simulink model "sldemo_mdlref_datamngt"  (R2019b)
settings: Solver=FixedStepDiscrete  StartTime=0.0  StopTime=10.0  RelTol=1e-3
PreLoadFcn:
  | sldemo_mdlref_datamngt_wsdata
  | sldemo_mdlref_counter_datamngt_types
undefined symbols (not defined in the file): CounterICs, CounterParams
settings Model: ModifiedByFormat=The MathWorks Inc.  ExtModeAutoUpdateStatusClock=off  Creator=The MathWorks, Inc.  LastModifiedBy=The MathWorks Inc.
settings DataIOCC: LimitDataPoints=on  SaveFormat=StructureWithTime  SaveOutput=off  SignalLogging=off  DSMLogging=off  SaveTime=off  ReturnWorkspaceOutputs=off  SignalLoggingName=logsOut
settings OptimizationCC: DefaultParameterBehavior=Inlined  InlineInvariantSignals=on  EnhancedBackFolding=on  StrengthReduction=on  ExpressionDepthLimit=2147483647  StateBitsets=on  DataBitsets=on  EfficientFloat2IntCast=on  LifeSpan=inf
settings DebuggingCC: SaveWithParameterizedLinksMsg=none  CheckExecutionContextPreStartOutputMsg=on  CheckExecutionContextRuntimeOutputMsg=on  MultiTaskDSMMsg=warning  MultiTaskCondExecSysMsg=none  SigSpecEnsureSampleTimeMsg=none  FcnCallInpInsideContextMsg=warning  StateNameClashWarn=warning  StrictBusMsg=ErrorOnBusTreatedAsVector  SFUnexpectedBacktrackingDiag=warning  SFNoUnconditionalDefaultTransitionDiag=warning  SFExecutionAtInitializationDiag=none  ArithmeticOperatorsInVariantConditions=warning
settings HardwareCC: ProdBitPerPointer=32  ProdBitPerSizeT=32  ProdBitPerPtrDiffT=32  ProdLargestAtomicFloat=None  ProdIntDivRoundTo=Undefined  ProdEndianess=Unspecified  ProdWordSize=32  ProdHWDeviceType=32-bit Generic  TargetHWDeviceType=32-bit Generic
settings ModelReferenceCC: UpdateModelReferenceTargets=IfOutOfDate  CheckModelReferenceTargetMessage=none  PropagateSignalLabelsOutOfModel=off
settings SFSimCC: SimUseLocalCustomCode=off  CustomCodeUndefinedFunction=UseInterfaceOnly
settings RTWCC: Description=Generic Real-Time Target  GenerateReport=on  RTWVerbose=off  RTWUseLocalCustomCode=off  LaunchReport=on
settings CodeAppCC: ForceParamTrailComments=on  MaxIdLength=100  StateflowObjectComments=on
settings GRTTargetCC: TargetLangStandard=C89/C90 (ANSI)  GeneratePreprocessorConditionals=Disable all  CombineOutputUpdateFcns=off  MatFileLogging=off  GRTInterface=on
settings ConfigComp: CovMetricSettings=dw  CovHtmlReporting=on  CovSaveCumulativeToWorkspaceVar=on  CovSaveSingleToWorkspaceVar=on  CovExternalEMLEnable=off  CovSFcnEnable=off

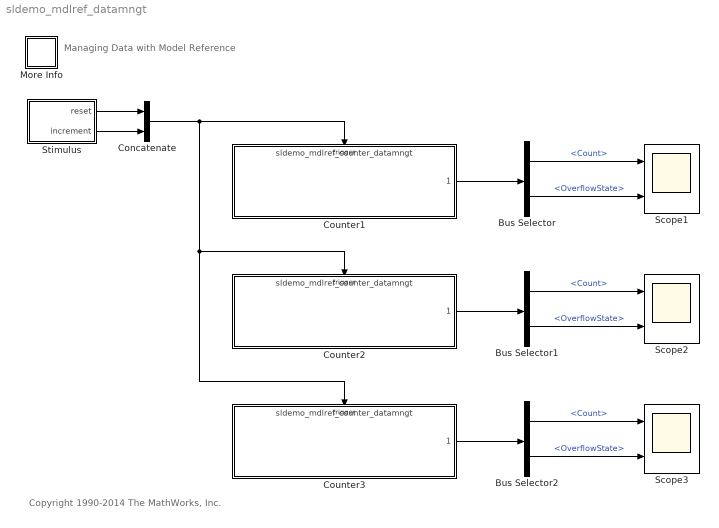
== system sldemo_mdlref_datamngt ==
  note: Managing Data with Model Reference
  note: Copyright 1990-2014 The MathWorks, Inc.
  Bus Selector : BusSelector  OutputSignals=Count,OverflowState
  Bus Selector1 : BusSelector  OutputSignals=Count,OverflowState
  Bus Selector2 : BusSelector  OutputSignals=Count,OverflowState
  Concatenate : Concatenate
  Counter1 : ModelReference  ModelNameDialog=sldemo_mdlref_counter_datamngt  ParameterArgumentNames=CounterICs,CounterParams  ParameterArgumentValues=CounterICs,CounterParams  UsingDefaultArgumentValue=0,0  ModelReferenceVersion=1.13  TriggerPortName=Trigger on rising edge  TriggerPortTriggerType=rising  CounterParams=Param1  CounterICs=IC1
  Counter2 : ModelReference  ModelNameDialog=sldemo_mdlref_counter_datamngt  ParameterArgumentNames=CounterICs,CounterParams  ParameterArgumentValues=CounterICs,CounterParams  UsingDefaultArgumentValue=0,0  ModelReferenceVersion=1.13  TriggerPortName=Trigger on rising edge  TriggerPortTriggerType=rising  CounterParams=Param2  CounterICs=IC1
  Counter3 : ModelReference  ModelNameDialog=sldemo_mdlref_counter_datamngt  ParameterArgumentNames=CounterICs,CounterParams  ParameterArgumentValues=CounterICs,CounterParams  UsingDefaultArgumentValue=0,0  ModelReferenceVersion=1.13  TriggerPortName=Trigger on rising edge  TriggerPortTriggerType=rising  CounterParams=Param2  CounterICs=IC2
  More Info : Subsystem
      settings: OpenFcn=showdemo(bdroot(gcb))
      mask Display: disp('?')
  Scope1 : Scope  NumInputPorts=2
  Scope2 : Scope  NumInputPorts=2
  Scope3 : Scope  NumInputPorts=2
  Stimulus : Subsystem  mask(Counter Input Stimulus){ResetPeriod=4, IncrementPeriod=0.2, SampleTime=0.1}
      mask prompts: ResetPeriod "Period for resetting counter:"; IncrementPeriod "Period for incrementing counter:"; SampleTime "Sample time:"
      mask help:
      | Provide input signals for driving counters.  Parameters control:
      | - The frequency of the input pulses to be counted.
      | - The frequency with which the counter should be reset.
  wires:
  Counter1/1 -> Bus Selector/1
  Bus Selector/1 -> Scope1/1  "<Count>"
  Bus Selector/2 -> Scope1/2  "<OverflowState>"
  Concatenate/1 -> Counter2/Trigger, Counter3/Trigger, Counter1/Trigger
  Counter2/1 -> Bus Selector1/1
  Bus Selector1/1 -> Scope2/1  "<Count>"
  Bus Selector1/2 -> Scope2/2  "<OverflowState>"
  Counter3/1 -> Bus Selector2/1
  Bus Selector2/1 -> Scope3/1  "<Count>"
  Bus Selector2/2 -> Scope3/2  "<OverflowState>"
  Stimulus/1(reset) -> Concatenate/1
  Stimulus/2(increment) -> Concatenate/2

== system sldemo_mdlref_datamngt/More Info ==
  note: This demonstration uses model arguments defined as parameter structures
      | to parameterize three instances of a referenced model that implements a
      | triggered counter algorithm.
  note: Bus Block Demonstration

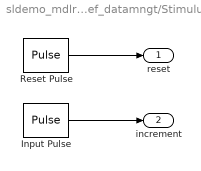
== system sldemo_mdlref_datamngt/Stimulus ==
  Input Pulse : DiscretePulseGenerator  Amplitude=logical(1)  Period=round(IncrementPeriod/SampleTime)  SampleTime=SampleTime  VectorParams1D=off
  Reset Pulse : DiscretePulseGenerator  Amplitude=logical(1)  Period=round(ResetPeriod/SampleTime)  SampleTime=SampleTime  VectorParams1D=off
  reset : Outport  VectorParamsAs1DForOutWhenUnconnected=off
  increment : Outport  Port=2  VectorParamsAs1DForOutWhenUnconnected=off
  wires:
  Input Pulse/1 -> increment/1
  Reset Pulse/1 -> reset/1
